simulink model "cukModelStateSpaceWithcontrol"  (R2020a)
settings: Solver=VariableStepAuto  StartTime=0.0  StopTime=0.3  RelTol=1e-9  AbsTol=4e-3
undefined symbols (not defined in the file): Asigma, b1, b2, bsigma, Csigma, Cxe, delta, f_s, fbounds, jthVec, Masigma, Mbsigma, Mcsigma, Nasigma, Nbsigma, Ncsigma, obsControl, obsSys, P, t_f, taua1, taua2, Tmax, uncertFreq, uncertType, x0, x_e, xe, xfdio0, xhat0
libraries: PhdLibrary x23, dspsigops x7, powerlib_meascontrol x5, dspmathops x1
(part 2 of 2)

== matlab function cukModelStateSpaceWithcontrol/Subsystem2/MATLAB Function ==
  data: t input; y output
function y = fcn(t)
% if (0<=t) && (t < 0.05)
%     y = 2-2*exp(-20*log(2)*sin(t));
% elseif (0.05<=t) && (t < 0.10)
%     y = 3*exp(-20*log(3)*(t-0.05))-2;
% elseif (0.10<=t) && (t < 0.15)
%     y = -3*exp(-20*log(3)*(t-0.15))-2;
%    % y = 1-2*exp(-20*log(2)*(t-0.1));
% else 
%     y = 0;
% end

y  = (2/pi)*asin(sin(60*t));
%y  = sin(t*30);
%y = sin(pi*t*100)*exp(-20*log(2)*t);
